simulink model "ZMP_preview_control"  (R2018b)
settings: Solver=ode15s  StartTime=0.0  StopTime=10  RelTol=1e-3
values from neighbouring files (symbols this model uses):
  arm_radius = leg_radius    (= 0.01)    [Nao_paramter.m]
  foot_height = 0.02    [Nao_paramter.m]
  foot_length = 0.1    [Nao_paramter.m]
  foot_mass = 0.17184    [Nao_paramter.m]
  foot_width = 0.05    [Nao_paramter.m]
  ground_height = 0.0025    [Nao_paramter.m]
  ground_length = 5    [Nao_paramter.m]
  ground_width = 2    [Nao_paramter.m]
  hand_mass = 0.18533    [Nao_paramter.m]
  head_mass = 0.60533    [Nao_paramter.m]
  hip_mass = 0.14053    [Nao_paramter.m]
  hip_off_Y = 0.05    [Nao_paramter.m]
  hip_off_Z = 0.085    [Nao_paramter.m]
  leg_radius = 0.01    [Nao_paramter.m]
  lowerarm_length = 0.05595    [Nao_paramter.m]
  lowerarm_mass = 0.07761    [Nao_paramter.m]
  neck_length = 0.03    [Nao_paramter.m]
  neck_mass = 0.07842    [Nao_paramter.m]
  neck_off_Z = 0.1265    [Nao_paramter.m]
  shoulder_mass = 0.09304    [Nao_paramter.m]
  thigh_mass = 0.38968    [Nao_paramter.m]
  tibia_mass = 0.30142    [Nao_paramter.m]
  torso_height = foot_height + tibia_length + thigh_length + 0.5*hip_off_Z    (= 0.2654)    [Nao_paramter.m]
  torso_mass = 1.0496    [Nao_paramter.m]
  upperarm_length = 0.105    [Nao_paramter.m]
  upperarm_mass = 0.15777    [Nao_paramter.m]
undefined symbols (not defined in the file or in its folder): Ad, Bd, Cd, DiscIntNeverNeededParam, sigbuilder_block, X, Y, Z
libraries: sm_lib x82, nesl_utility x15, Contact_Forces_Lib x10
(part 4 of 4)

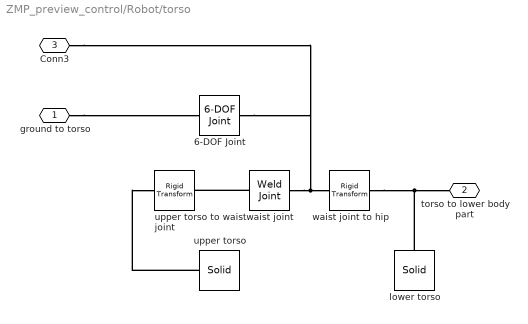
== system ZMP_preview_control/Robot/torso ==
  " waist joint" : sm_lib/Joints/Weld Joint  SenseConstraintForce=off  SenseConstraintForceX=off  SenseConstraintForceY=off  SenseConstraintForceZ=off  SenseConstraintTorque=off  SenseConstraintTorqueX=off  SenseConstraintTorqueY=off  SenseConstraintTorqueZ=off  SenseTotalForce=off  SenseTotalForceX=off  SenseTotalForceY=off  SenseTotalForceZ=off  SenseTotalTorque=off  SenseTotalTorqueX=off  SenseTotalTorqueY=off  SenseTotalTorqueZ=off  CompositeWrenchDir=FollowerOnBase  CompositeWrenchFrame=BaseFrame
  6-DOF Joint : sm_lib/Joints/6-DOF Joint  SenseConstraintForce=off  SenseConstraintForceX=off  SenseConstraintForceY=off  SenseConstraintForceZ=off  SenseConstraintTorque=off  SenseConstraintTorqueX=off  SenseConstraintTorqueY=off  SenseConstraintTorqueZ=off  SenseTotalForce=off  SenseTotalForceX=off  SenseTotalForceY=off  SenseTotalForceZ=off  SenseTotalTorque=off  SenseTotalTorqueX=off  SenseTotalTorqueY=off  SenseTotalTorqueZ=off  CompositeWrenchDir=FollowerOnBase  CompositeWrenchFrame=BaseFrame  PxEquilibriumPosition=0  PxEquilibriumPositionUnits=m  PxSpringStiffness=1000  PxSpringStiffnessUnits=N/m  PxDampingCoefficient=800  PxDampingCoefficientUnits=N/(m/s)  PxTorqueActuationMode=NoTorque  PxMotionActuationMode=ComputedMotion  PxSensePosition=off  PxSenseVelocity=off  PxSenseAcceleration=off  PxSenseTorqueForce=off  PxPositionTargetSpecify=on  PxPositionTargetPriority=High  PxPositionTargetValue=0  PxPositionTargetValueUnits=m  PxVelocityTargetSpecify=off  PxVelocityTargetPriority=High  PxVelocityTargetValue=0  PxVelocityTargetValueUnits=m/s  PyEquilibriumPosition=0  PyEquilibriumPositionUnits=m  PySpringStiffness=1000  PySpringStiffnessUnits=N/m  PyDampingCoefficient=800  PyDampingCoefficientUnits=N/(m/s)  PyTorqueActuationMode=NoTorque  PyMotionActuationMode=ComputedMotion  PySensePosition=off  PySenseVelocity=off  PySenseAcceleration=off  PySenseTorqueForce=off  PyPositionTargetSpecify=on  PyPositionTargetPriority=High  PyPositionTargetValue=0  PyPositionTargetValueUnits=m  PyVelocityTargetSpecify=off  PyVelocityTargetPriority=High  PyVelocityTargetValue=0  PyVelocityTargetValueUnits=m/s  PzEquilibriumPosition=0  PzEquilibriumPositionUnits=m  PzSpringStiffness=1000  PzSpringStiffnessUnits=N/m  PzDampingCoefficient=800  PzDampingCoefficientUnits=N/(m/s)  PzTorqueActuationMode=NoTorque  PzMotionActuationMode=ComputedMotion  PzSensePosition=off  PzSenseVelocity=off  PzSenseAcceleration=off  PzSenseTorqueForce=off  PzPositionTargetSpecify=on  PzPositionTargetPriority=High  PzPositionTargetValue=torso_height+0.001  PzPositionTargetValueUnits=m  PzVelocityTargetSpecify=off  PzVelocityTargetPriority=High  PzVelocityTargetValue=0  PzVelocityTargetValueUnits=m/s  SphDefPosRotationMethod=None  SphDefPosRotationAngleUnits=deg  SphDefPosRotationStandardAxis=+Z  SphDefPosRotationAngle=0.0  SphDefPosRotationArbitraryAxis=[0 0 1]  SphDefPosFollAlignAxisA=+X  SphDefPosBaseAlignAxisA=+Y  SphDefPosFollAlignAxisB=+Y  SphDefPosBaseAlignAxisB=+Z  SphDefPosRotationSequenceAxes=FollowerAxes  SphDefPosRotationSequence=XYX  SphDefPosRotationSequenceAngles=[0 0 0]  SphDefPosRotationSequenceAnglesUnits=deg  SphDefPosRotationMatrix=[1 0 0; 0 1 0; 0 0 1]  SphEqPosRotationMethod=None  SphEqPosRotationAngleUnits=deg  SphEqPosRotationStandardAxis=+Z  SphEqPosRotationAngle=0.0  SphEqPosRotationArbitraryAxis=[0 0 1]  SphEqPosFollAlignAxisA=+X  SphEqPosBaseAlignAxisA=+Y  SphEqPosFollAlignAxisB=+Y  SphEqPosBaseAlignAxisB=+Z  SphEqPosRotationSequenceAxes=FollowerAxes  SphEqPosRotationSequence=XYX  SphEqPosRotationSequenceAngles=[0 0 0]  SphEqPosRotationSequenceAnglesUnits=deg  SphEqPosRotationMatrix=[1 0 0; 0 1 0; 0 0 1]  SphSpringStiffness=1000  SphSpringStiffnessUnits=N*m/deg  SphDampingCoefficient=1000  SphDampingCoefficientUnits=N*m/(rad/s)  SphActuateTorqueX=off  SphActuateTorqueY=off  SphActuateTorqueZ=off  SphActuateTorque=off  SphTorqueActuationMode=NoTorque  SphMotionActuationMode=ComputedMotion  SphActuationFrame=BaseFrame  SphSensePosition=off  SphSenseVelocityX=off  SphSenseVelocityY=off  SphSenseVelocityZ=off  SphSenseVelocity=off  SphSenseAccelerationX=off  SphSenseAccelerationY=off  SphSenseAccelerationZ=off  SphSenseAcceleration=off  SphSenseTorqueX=off  SphSenseTorqueY=off  SphSenseTorqueZ=off  SphSenseTorqueForce=off  SphSensingFrame=BaseFrame  SphPositionTargetRotationMethod=None  SphPositionTargetRotationAngleUnits=deg  SphPositionTargetRotationStandardAxis=+Z  SphPositionTargetRotationAngle=0.0  SphPositionTargetRotationArbitraryAxis=[0 0 1]  SphPositionTargetFollAlignAxisA=+X  SphPositionTargetBaseAlignAxisA=+Y  SphPositionTargetFollAlignAxisB=+Y  SphPositionTargetBaseAlignAxisB=+Z  SphPositionTargetRotationSequenceAxes=FollowerAxes  SphPositionTargetRotationSequence=XYX  SphPositionTargetRotationSequenceAngles=[0 0 0]  SphPositionTargetRotationSequenceAnglesUnits=deg  SphPositionTargetRotationMatrix=eye(3)  SphPositionTargetSpecify=off  SphPositionTargetPriority=High  SphVelocityTargetValue=[0 0 0]  SphVelocityTargetValueUnits=deg/s  SphVelocityTargetSpecify=off  SphVelocityTargetPriority=High  SphVelocityTargetInFollowerFrame=on
  lower torso : sm_lib/Body Elements/Solid  InertiaType=CalculateFromGeometry  Mass=hip_mass  MassUnits=kg  CenterOfMass=[0 0 0]  CenterOfMassUnits=m  MomentsOfInertia=[1 1 1]  MomentsOfInertiaUnits=kg*m^2  ProductsOfInertia=[1 1 1]  ProductsOfInertiaUnits=kg*m^2  BasedOnType=Mass  Density=1000  DensityUnits=kg/m^3  DoExposeReferenceFrame=on  SerializedFrames=<Frames/>  GraphicType=FromGeometry  MarkerShape=Sphere  MarkerSize=10  GraphicVisPropType=SimpleVisualProperties  GraphicDiffuseColor=[0.6 0.6 0.6]  GraphicSpecularColor=[0.5 0.5 0.5 1.0]  GraphicAmbientColor=[0.15 0.15 0.15 1.0]  GraphicEmissiveColor=[0.0 0.0 0.0 1.0]  GraphicShininess=75  GraphicOpacity=1.0  GeometryShape=Brick  RectangleSize=[1 1]  RectangleSizeUnits=m  BrickDimensions=[0.5*foot_length 2*hip_off_Y hip_off_Z]  BrickDimensionUnits=m  CylinderRadius=1  CylinderRadiusUnits=m  CylinderLength=1  CylinderLengthUnits=m  SphereRadius=1  SphereRadiusUnits=m  EllipsoidRadii=[1 1 1]  EllipsoidRadiiUnits=m  ExtrusionCrossSection=[1 1; -1 1; -1 -1; 1 -1]  ExtrusionCrossSectionUnits=m  ExtrusionLength=1  ExtrusionLengthUnits=m  PolygonNumSides=3  PolygonOuterRadius=1  PolygonOuterRadiusUnits=m  ExtGeomFileType=STEP  ExtGeomFileUnits=m  RevolutionCrossSection=[1 1; 1 -1; 2 -1; 2 1]  RevolutionCrossSectionUnits=m  RevolutionExtent=Full  RevolutionAngle=180  RevolutionAngleUnits=deg
  upper torso : sm_lib/Body Elements/Solid  InertiaType=Custom  Mass=torso_mass  MassUnits=kg  CenterOfMass=[-0.00413 0 0.5*neck_off_Z]  CenterOfMassUnits=m  MomentsOfInertia=torso_inertia_m  MomentsOfInertiaUnits=kg*m^2  ProductsOfInertia=torso_inertia_p  ProductsOfInertiaUnits=kg*m^2  BasedOnType=Mass  Density=1000  DensityUnits=kg/m^3  DoExposeReferenceFrame=on  SerializedFrames=<Frames/>  GraphicType=FromGeometry  MarkerShape=Sphere  MarkerSize=10  GraphicVisPropType=SimpleVisualProperties  GraphicDiffuseColor=[0.5 0.5 0.5]  GraphicSpecularColor=[0.5 0.5 0.5 1.0]  GraphicAmbientColor=[0.15 0.15 0.15 1.0]  GraphicEmissiveColor=[0.0 0.0 0.0 1.0]  GraphicShininess=75  GraphicOpacity=1.0  GeometryShape=Brick  RectangleSize=[1 1]  RectangleSizeUnits=m  BrickDimensions=[2*hip_off_Y 2.5*foot_width neck_off_Z]  BrickDimensionUnits=m  CylinderRadius=1  CylinderRadiusUnits=m  CylinderLength=1  CylinderLengthUnits=m  SphereRadius=1  SphereRadiusUnits=m  EllipsoidRadii=[1 1 1]  EllipsoidRadiiUnits=m  ExtrusionCrossSection=[1 1; -1 1; -1 -1; 1 -1]  ExtrusionCrossSectionUnits=m  ExtrusionLength=1  ExtrusionLengthUnits=m  PolygonNumSides=3  PolygonOuterRadius=1  PolygonOuterRadiusUnits=m  ExtGeomFileType=STEP  ExtGeomFileUnits=m  RevolutionCrossSection=[1 1; 1 -1; 2 -1; 2 1]  RevolutionCrossSectionUnits=m  RevolutionExtent=Full  RevolutionAngle=180  RevolutionAngleUnits=deg
  upper torso to waist joint : sm_lib/Frames and Transforms/Rigid Transform  TranslationMethod=StandardAxis  TranslationStandardOffset=0.5*neck_off_Z  TranslationLengthUnit=m  TranslationStandardAxis=-Z  TranslationCartesianOffset=[0 0 0]  TranslationROffset=0  TranslationROffsetUnits=m  TranslationZOffset=0  TranslationZOffsetUnits=m  TranslationThetaOffset=0  TranslationThetaOffsetUnits=deg  RotationMethod=None  RotationAngleUnits=deg  RotationStandardAxis=+Z  RotationAngle=0.0  RotationArbitraryAxis=[0 0 1]  FollAlignAxisA=+X  BaseAlignAxisA=+Y  FollAlignAxisB=+Y  BaseAlignAxisB=+Z  RotationSequenceAxes=FollowerAxes  RotationSequence=XYX  RotationSequenceAngles=[0 0 0]  RotationSequenceAnglesUnits=deg  RotationMatrix=[1 0 0; 0 1 0; 0 0 1]
  waist joint to hip : sm_lib/Frames and Transforms/Rigid Transform  TranslationMethod=StandardAxis  TranslationStandardOffset=0.5*hip_off_Z  TranslationLengthUnit=m  TranslationStandardAxis=-Z  TranslationCartesianOffset=[0 0 0]  TranslationROffset=0  TranslationROffsetUnits=m  TranslationZOffset=0  TranslationZOffsetUnits=m  TranslationThetaOffset=0  TranslationThetaOffsetUnits=deg  RotationMethod=None  RotationAngleUnits=deg  RotationStandardAxis=+Z  RotationAngle=0.0  RotationArbitraryAxis=[0 0 1]  FollAlignAxisA=+X  BaseAlignAxisA=+Y  FollAlignAxisB=+Y  BaseAlignAxisB=+Z  RotationSequenceAxes=FollowerAxes  RotationSequence=XYX  RotationSequenceAngles=[0 0 0]  RotationSequenceAnglesUnits=deg  RotationMatrix=[1 0 0; 0 1 0; 0 0 1]
  ground to torso : PMIOPort  Side=Left
  torso to lower body part : PMIOPort  Port=2  Side=Right
  Conn3 : PMIOPort  Port=3  Side=Left
  connections:
  upper torso/RConn1 -- upper torso to waist joint/LConn1
  " waist joint"/RConn1 -- 6-DOF Joint/RConn1 -- Conn3/RConn1 -- waist joint to hip/LConn1
  waist joint to hip/RConn1 -- lower torso/RConn1 -- torso to lower body part/RConn1
  " waist joint"/LConn1 -- upper torso to waist joint/RConn1
  ground to torso/RConn1 -- 6-DOF Joint/LConn1

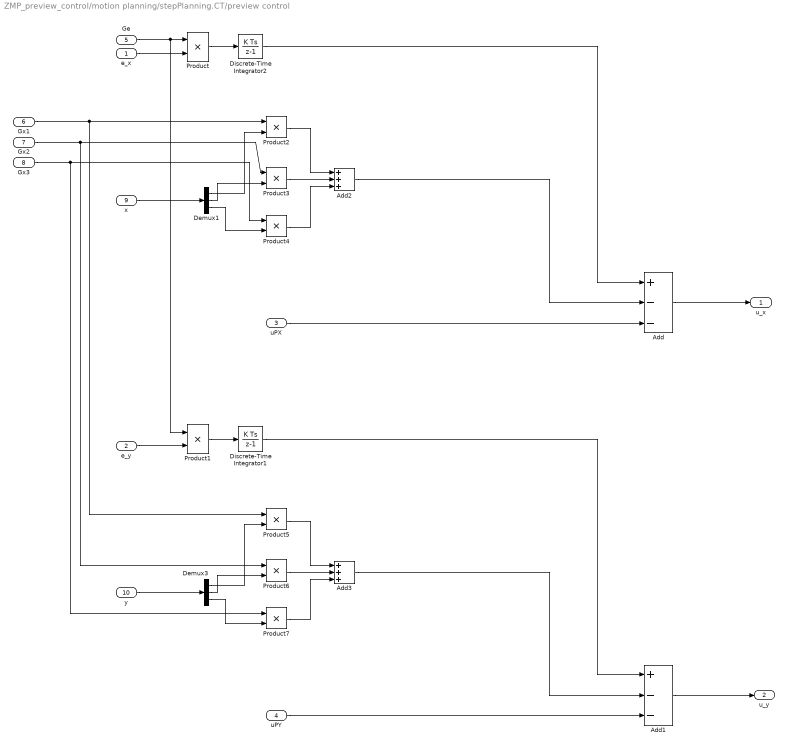
== system ZMP_preview_control/motion planning/stepPlanning.CT/preview control ==
  e_x : Inport  OutDataTypeStr=double
  e_y : Inport  Port=2  OutDataTypeStr=double  PortDimensions=1
  uPX : Inport  Port=3  OutDataTypeStr=double  PortDimensions=1
  uPY : Inport  Port=4  OutDataTypeStr=double  PortDimensions=1
  Ge : Inport  Port=5  OutDataTypeStr=double
  Gx1 : Inport  Port=6  OutDataTypeStr=double  PortDimensions=1
  Gx2 : Inport  Port=7  OutDataTypeStr=double  PortDimensions=1
  Gx3 : Inport  Port=8  OutDataTypeStr=double  PortDimensions=1
  x : Inport  Port=9  OutDataTypeStr=double  PortDimensions=[3 1]
  y : Inport  Port=10  OutDataTypeStr=double  PortDimensions=[3 1]
  Add : Sum  Inputs=+--
  Add1 : Sum  Inputs=+--
  Add2 : Sum  Inputs=3
  Add3 : Sum  Inputs=3
  Demux1 : Demux  Outputs=3
  Demux3 : Demux  Outputs=3
  Discrete-Time Integrator1 : DiscreteIntegrator  gainval=1  SampleTime=-1  OutDataTypeStr=double  ICPrevOutput=DiscIntNeverNeededParam  ICPrevScaledInput=DiscIntNeverNeededParam
  Discrete-Time Integrator2 : DiscreteIntegrator  gainval=1  SampleTime=-1  OutDataTypeStr=double  ICPrevOutput=DiscIntNeverNeededParam  ICPrevScaledInput=DiscIntNeverNeededParam
  Product : Product  OutDataTypeStr=double
  Product1 : Product  OutDataTypeStr=double
  Product{2..7} (6 alike) : Product
  u_x : Outport  OutDataTypeStr=double  PortDimensions=1
  u_y : Outport  Port=2  OutDataTypeStr=double  PortDimensions=1
  wires:
  e_x/1 -> Product/2
  Product/1 -> Discrete-Time Integrator2/1
  Add/1 -> u_x/1
  Ge/1 -> Product1/1, Product/1
  x/1 -> Demux1/1
  Demux1/1 -> Product2/2
  Demux1/2 -> Product3/2
  Demux1/3 -> Product4/2
  Product2/1 -> Add2/1
  Product3/1 -> Add2/2
  Product4/1 -> Add2/3
  uPX/1 -> Add/3
  Add2/1 -> Add/2
  Discrete-Time Integrator2/1 -> Add/1
  Product6/1 -> Add3/2
  Product5/1 -> Add3/1
  Demux3/3 -> Product7/2
  Demux3/1 -> Product5/2
  Gx1/1 -> Product5/1, Product2/1
  y/1 -> Demux3/1
  Product7/1 -> Add3/3
  Discrete-Time Integrator1/1 -> Add1/1
  e_y/1 -> Product1/2
  Gx3/1 -> Product7/1, Product4/1
  Product1/1 -> Discrete-Time Integrator1/1
  Add3/1 -> Add1/2
  Gx2/1 -> Product6/1, Product3/1
  Demux3/2 -> Product6/2
  Add1/1 -> u_y/1
  uPY/1 -> Add1/3

== stateflow chart ZMP_preview_control/motion planning ==
  state stepPlanning
    entry:
    time = 30;
    hipOff = 0.05;
    sD = 0.2;         % second
    sStr = 0.03;       % forward step size
    sSi = 0.05;        % sideward step size
    H = 0.01;            % foot lifting height
    [zmpX,zmpY,uPX,uPY,gainE,gainX] = gen(sD,sStr,hipOff,time);
    CoMX = zeros(1,time*100+1);
    CoMY = zeros(1,time*100+1);
    k = 0;
    state CoMGen1
      entry:
      k = k+1;
      zmpXk = zmpX(k);
      zmpYk = zmpY(k);
      uPXk = uPX(k);
      uPYk = uPY(k);
      [CoMXk,CoMYk] = CT(zmpXk,zmpYk,uPXk,uPYk,gainE,gainX);
      CoMX(:,k) = CoMXk;
      CoMY(:,k) = CoMYk;
    state [comx,comy] = CT(zmpx,zmpy,ux,uy,Ge,Gx) [function]
    state motionGenR
      entry:
      [hRor,hRol,hPir,hPil,hYar,hYal,kBer,kBel,aRor,aRol,aPir,aPil]=motionR(sD,sStr,sSi,H,CoMX,CoMY);
      state outR
        entry:
        j = j+1;
        hipRollR = hRor(j);
        hipRollL = hRol(j);
        hipPitchR = hPir(j);
        hipPitchL = hPil(j);
        hipYawR = hYar(j);
        hipYawL = hYal(j);
        kneeBendR = kBer(j);
        kneeBendL = kBel(j);
        ankleRollR = aRor(j);
        ankleRollL = aRol(j);
        anklePitchR = aPir(j);
        anklePitchL = aPil(j);
      (default) -> outR : {j = 0;}
      outR -> outR : after(sD/100,sec)
    state motionGenL
      entry:
      [hRor,hRol,hPir,hPil,hYar,hYal,kBer,kBel,aRor,aRol,aPir,aPil]=motionL(sD,sStr,sSi,H,CoMX,CoMY);
      state outL
        entry:
        j = j+1;
        hipRollR = hRor(j);
        hipRollL = hRol(j);
        hipPitchR = hPir(j);
        hipPitchL = hPil(j);
        hipYawR = hYar(j);
        hipYawL = hYal(j);
        kneeBendR = kBer(j);
        kneeBendL = kBel(j);
        ankleRollR = aRor(j);
        ankleRollL = aRol(j);
        anklePitchR = aPir(j);
        anklePitchL = aPil(j);
      (default) -> outL : {j = 0;}
      outL -> outL : after(sD/100,sec)
    (junction 536) -> CoMGen1 [order 1] : [k < (time*100+1)]
    (default) -> CoMGen1
    CoMGen1 -> (junction 536)
    (junction 536) -> motionGenL [order 2] : [(k >= (time*100+1)) ]
    motionGenL -> motionGenR : [j > 99]
    motionGenR -> motionGenL : [j > 99]
  (default) -> stepPlanning
  data: zmpx function_input double size=1; zmpy function_input double size=1; ux function_input double size=1; uy function_input double size=1; Ge function_input double size=1; Gx function_input double size=[3 1]; comx function_output; comy function_output double size=1; stepDuration function_input; stepStraight function_input; zmp function_input; X function_output; Y function_output; uX function_output; uY function_output; Ge function_output; Gx function_output; t function_input; hRr function_output; hRl function_output; hPr function_output; hPl function_output; hYr function_output; hYl function_output; kBr function_output; kBl function_output; aRr function_output; aRl function_output; aPr function_output; aPl function_output; stepDuration function_input; stepStr function_input; stepSide function_input; liftH function_input; comx function_input; comy function_input; hRr function_output; hRl function_output; hPr function_output; hPl function_output; hYr function_output; hYl function_output; kBr function_output; kBl function_output; aRr function_output; aRl function_output; aPr function_output; aPl function_output; stepDuration function_input; stepStr function_input; stepSide function_input; liftH function_input; comx function_input; comy function_input; hipRollL output; hipRollR output; hipPitchL output; hipPitchR output; hipYawL output; hipYawR output; kneeBendL output; kneeBendR output; k local double size=1; ankleRollL output; ankleRollR output; anklePitchL output; anklePitchR output; aPil local; aPir local; aRol local; aRor local; hPil local; hPir local; hRol local; hRor local; hYal local; hYar local; kBel local; kBer local; H local; sD local; sSi local; sStr local; zmpX local double size=[1 3001]; zmpY local size=[1 3001]; hipOff local; zmpXk local double size=1; zmpYk local double size=1; uPX local size=[1 3001]; uPY local size=[1 3001]; gainE local size=1; gainX local size=[3 1]; uPXk local; uPYk local; time local; j local; CoMXk local size=1; CoMYk local size=1; l local; CoMX local size=[1 3001]; CoMY local size=[1 3001]
  function [X,Y,uX,uY,Ge,Gx] = gen(stepDuration,stepStraight,zmp,t):
    | function [X,Y,uX,uY,Ge,Gx] = gen(stepDuration,stepStraight,zmp,t)
    | time = t;
    | t = 0:0.01:time;
    | tt = 0:0.01:stepDuration;
    | tt1 = stepDuration*[0 0.25 0.5 0.75 1];
    | %% zmp y
    | begY = pchip(tt1,[0 0 0 0 -zmp],tt);
    | NY = (time-2*stepDuration)/(2*stepDuration);
    | cycleYD = pchip(tt1,[zmp zmp zmp zmp zmp],tt);
    | cycleYD(:,1) = [];
    | cycleYU = pchip(tt1,[-zmp -zmp -zmp -zmp -zmp],tt);
    | cycleYU(:,1) = [];
    | cycleY = [cycleYD cycleYU];
    | endY = pchip(tt1,[-zmp -zmp -zmp -zmp -zmp],tt);
    | endY(:,1) = [];
    | Y = [begY repmat(cycleY,1,NY) endY];
    | 
    | %% zmp x
    | NX = time/stepDuration-1;
    | zmpXX = zeros(NX+1,length(t));
    | for i = 2:NX-1
    |     zmpXX(i+2,:) = stepStraight*ones(1,length(t));
    |     zmpXX(i+2,1:i*length(tt)-i+1) = zeros(1,i*length(tt)-i+1);
    | end
    | X = sum(zmpXX);
    | 
    | %% ZMP preview
    | coder.extrinsic('dare');
    | Ad = [1 0.01 5e-5;0 1 0.01;0 0 1];
    | Bd = [1.6667e-7;5e-05;0.01];
    | Cd = [1 0 -0.0296];
    | Dd = 0;
    | 
    | N = 50;
    | Qe = 1000;
    | Qx = [0 0 0;0 0 0;0 0 0];
    | R = 0.6;
    | B_til = [Cd*Bd;Bd];
    | F_til = [Cd*Ad;Ad];
    | I_til = [1 zeros(1,3)]';
    | A_til = [I_til F_til];
    | A_ctil = zeros(4,4);
    | K_til = zeros(4,4);
    | Q_til = [Qe zeros(1,3);zeros(3,1) Qx];
    | [K_til,L,G] = dare(A_til,B_til,Q_til,R);
    | A_ctil = A_til-B_til*(R+B_til'*K_til*B_til)'*B_til'*K_til*A_til;
    | Ge = (R+B_til'*K_til*B_til)\B_til'*K_til*I_til;
    | Gx = ((R+B_til'*K_til*B_til)\B_til'*K_til*F_til)';
    | uX = zeros(1,size(X,2));
    | uY = zeros(1,size(Y,2));
    | Gp = zeros(1,N);
    | X_til = zeros(4,N);
    | %%
    | for k = 1:size(X(1,:),2)
    |     temp1_x = 0;
    |     if ((k+N) < size(X(1,:),2))
    |         for l = 1:N
    |             if l == 1
    |                 X_til(:,1) = -A_ctil'*K_til*I_til;
    |                 Gp(l) = -Ge;
    |             elseif l >= 2
    |                 Gp(l) = (R+B_til'*K_til*B_til)\B_til'*X_til(:,l-1);
    |                 X_til(:,l) = A_ctil'*X_til(:,l-1); 
    |             end
    |             temp1_x = temp1_x + Gp(l)*X(1,k+l);
    |         end
    |         uX(k) = temp1_x;
    |     else
    |         uX(k) = uX(k-1);
    |     end
    | end
    | 
    | % Right foot y direction
    | for k = 1:size(Y(1,:),2)
    |     temp1_y = 0;
    |     if ((k+N) <= size(Y(1,:),2))
    |         for l = 1:N
    |             if l == 1
    |                 X_til(:,1) = -A_ctil'*K_til*I_til;
    |                 Gp(l) = -Ge;
    |             elseif l >= 2
    |                 Gp(l) = (R+B_til'*K_til*B_til)\B_til'*X_til(:,l-1);
    |                 X_til(:,l) = A_ctil'*X_til(:,l-1); 
    |             end
    |             temp1_y = temp1_y + Gp(l)*Y(1,k+l);
    |         end
    |         uY(k) = temp1_y;
    |     else
    |         uY(k) = uY(k-1);
    |     end
    | end
  function [hRr,hRl,hPr,hPl,hYr,hYl,kBr,kBl,aRr,aRl,aPr,aPl] = motionL(stepDuration,stepStr,...:
    | function [hRr,hRl,hPr,hPl,hYr,hYl,kBr,kBl,aRr,aRl,aPr,aPl] = motionL(stepDuration,stepStr,...
    |     stepSide,liftH,comx,comy)
    | CoMOffx = 0.05;  
    | CoMOffy = -0.0084;%max(comy(:,1500:1600));
    | t = linspace(0,stepDuration,100);
    | 
    | L = 0.2029;
    | tt = stepDuration*[0 0.1 0.2 0.3 0.4 0.5 0.6 0.7 0.8 0.9 1];
    | % hip roll
    | hR1 = pi/2-acos(CoMOffy*sin(pi/stepDuration*tt(:,1))/L);
    | hR2 = pi/2-acos(CoMOffy*sin(pi/stepDuration*tt(:,4))/L);
    | hR3 = pi/2-acos(CoMOffy*sin(pi/stepDuration*tt(:,6))/L);
    | hR4 = pi/2-acos(CoMOffy*sin(pi/stepDuration*tt(:,8))/L);
    | hR5 = pi/2-acos(CoMOffy*sin(pi/stepDuration*tt(:,11))/L);
    | 
    | hRl = -pchip([tt(:,1),tt(:,4),tt(:,6),tt(:,8),tt(:,11)],[hR1,hR2,hR3,hR4,hR5],t);
    | hRr = hRl;
    | % left hip pitch
    | hPl1 = 0;
    | hPl2 = asin(stepStr*sin(pi/stepDuration*tt(:,4))/sqrt((L*cos(hR2)-liftH)^2+...
    |     (stepStr*sin(pi/stepDuration*tt(:,4)))^2))+acos((0.1^2+(L*cos(hR2)-liftH)^2+...
    |     (stepStr*sin(pi/stepDuration*tt(:,4)))^2-0.1029^2)/(2*0.1*sqrt((L*cos(hR2)-liftH)^2+...
    |     (stepStr*sin(pi/stepDuration*tt(:,4)))^2)));
    | hPl3 = acos(((L*cos(hR3))^2+L^2-stepStr^2)/(2*L*cos(hR3)*L));
    | hPl4 = acos(((L*cos(hR4))^2+L^2-(stepStr*sin(pi/stepDuration*tt(:,8)))^2)/...
    |     (2*(L*cos(hR4))*L));
    | hPl5 = 0;
    | hPl = -pchip([tt(:,1),tt(:,4),tt(:,6),tt(:,8),tt(:,11)],[hPl1,hPl2,hPl3,hPl4,hPl5],t);
    | % right hip pitch
    | hPr1 = 0;
    | hPr2 = atan(CoMOffx*sin(pi/stepDuration*tt(:,4))/(L*cos(hR2)));
    | hPr3 = atan(CoMOffx/(L*cos(hR3)));
    | hPr4 = atan(CoMOffx*sin(pi/stepDuration*tt(:,8))/(L*cos(hR2)));
    | hPr5 = 0;
    | hPr = pchip([tt(:,1),tt(:,4),tt(:,6),tt(:,8),tt(:,11)],[hPr1,hPr2,hPr3,hPr4,hPr5],t);
    | % right hip yaw
    | hYr = pchip([tt(:,1),tt(:,4),tt(:,6),tt(:,8),tt(:,11)],[0 0 0 0 0],t);
    | % left hip yaw
    | hYl = pchip([tt(:,1),tt(:,4),tt(:,6),tt(:,8),tt(:,11)],[0 0 0 0 0],t);
    | % right knee bend
    | kBl1 = -0.15;
    | kBl2 = -pi+acos((0.1^2+0.1029^2-(L*cos(hR2)-liftH)^2-...
    |     (stepStr*sin(pi/stepDuration*tt(:,4)))^2)/(2*0.1*0.1029));
    | kBl3 = 0;
    | kBl4 = 0;
    | kBl5 = 0;
    | kBl = pchip([tt(:,1),tt(:,4),tt(:,6),tt(:,8),tt(:,11)],[kBl1,kBl2,kBl3,kBl4,kBl5],t);
    | % left knee bend
    | kBr = pchip([tt(:,1),tt(:,4),tt(:,6),tt(:,8),tt(:,11)],[-0.15 -0.15 -0.15 -0.15 -0.15],t);
    | % right angle pitch 
    | aPr = -hPr+kBr;
    | % left ankle pitch
    | aPl = -hPl+kBl;
    | % right ankle roll
    | aRl = -hRl;
    | % left ankle roll
    | aRr = -hRr;
  function [hRr,hRl,hPr,hPl,hYr,hYl,kBr,kBl,aRr,aRl,aPr,aPl] = motionR(stepDuration,stepStr,...:
    | function [hRr,hRl,hPr,hPl,hYr,hYl,kBr,kBl,aRr,aRl,aPr,aPl] = motionR(stepDuration,stepStr,...
    |     stepSide,liftH,comx,comy)
    | CoMOffx = 0.05;  
    | CoMOffy = 0.0084;%max(comy(:,1500:1600));
    | t = linspace(0,stepDuration,100);
    | 
    | L = 0.2029;
    | tt = stepDuration*[0 0.1 0.2 0.3 0.4 0.5 0.6 0.7 0.8 0.9 1];
    | % hip roll
    | hR1 = pi/2-acos(CoMOffy*sin(pi/stepDuration*tt(:,1))/L);
    | hR2 = pi/2-acos(CoMOffy*sin(pi/stepDuration*tt(:,4))/L);
    | hR3 = pi/2-acos(CoMOffy*sin(pi/stepDuration*tt(:,6))/L);
    | hR4 = pi/2-acos(CoMOffy*sin(pi/stepDuration*tt(:,8))/L);
    | hR5 = pi/2-acos(CoMOffy*sin(pi/stepDuration*tt(:,11))/L);
    | 
    | hRl = -pchip([tt(:,1),tt(:,4),tt(:,6),tt(:,8),tt(:,11)],[hR1,hR2,hR3,hR4,hR5],t);
    | hRr = hRl;
    | % left hip pitch
    | hPr1 = 0;
    | hPr2 = asin(stepStr*sin(pi/stepDuration*tt(:,4))/sqrt((L*cos(hR2)-liftH)^2+...
    |     (stepStr*sin(pi/stepDuration*tt(:,4)))^2))+acos((0.1^2+(L*cos(hR2)-liftH)^2+...
    |     (stepStr*sin(pi/stepDuration*tt(:,4)))^2-0.1029^2)/(2*0.1*sqrt((L*cos(hR2)-liftH)^2+...
    |     (stepStr*sin(pi/stepDuration*tt(:,4)))^2)));
    | hPr3 = acos(((L*cos(hR3))^2+L^2-stepStr^2)/(2*L*cos(hR3)*L));
    | hPr4 = acos(((L*cos(hR4))^2+L^2-(stepStr*sin(pi/stepDuration*tt(:,8)))^2)/...
    |     (2*(L*cos(hR4))*L));
    | hPr5 = 0;
    | hPr = -pchip([tt(:,1),tt(:,4),tt(:,6),tt(:,8),tt(:,11)],[hPr1,hPr2,hPr3,hPr4,hPr5],t);
    | % right hip pitch
    | hPl1 = 0;
    | hPl2 = atan(CoMOffx*sin(pi/stepDuration*tt(:,4))/(L*cos(hR2)));
    | hPl3 = atan(CoMOffx/(L*cos(hR3)));
    | hPl4 = atan(CoMOffx*sin(pi/stepDuration*tt(:,8))/(L*cos(hR2)));
    | hPl5 = 0;
    | hPl = pchip([tt(:,1),tt(:,4),tt(:,6),tt(:,8),tt(:,11)],[hPl1,hPl2,hPl3,hPl4,hPl5],t);
    | % right hip yaw
    | hYr = pchip([tt(:,1),tt(:,4),tt(:,6),tt(:,8),tt(:,11)],[0 0 0 0 0],t);
    | % left hip yaw
    | hYl = pchip([tt(:,1),tt(:,4),tt(:,6),tt(:,8),tt(:,11)],[0 0 0 0 0],t);
    | % right knee bend
    | kBr1 = -0.15;
    | kBr2 = -pi+acos((0.1^2+0.1029^2-(L*cos(hR2)-liftH)^2-...
    |     (stepStr*sin(pi/stepDuration*tt(:,4)))^2)/(2*0.1*0.1029));
    | kBr3 = 0;
    | kBr4 = 0;
    | kBr5 = 0;
    | kBr = pchip([tt(:,1),tt(:,4),tt(:,6),tt(:,8),tt(:,11)],[kBr1,kBr2,kBr3,kBr4,kBr5],t);
    | % left knee bend
    | kBl = pchip([tt(:,1),tt(:,4),tt(:,6),tt(:,8),tt(:,11)],[-0.15 -0.15 -0.15 -0.15 -0.15],t);
    | % right angle pitch 
    | aPr = -hPr+kBr;
    | % left ankle pitch
    | aPl = -hPl+kBl;
    | % right ankle roll
    | aRl = -hRl;
    | % left ankle roll
    | aRr = -hRr;
